simulink model "first"  (R2020b)
settings: Solver=VariableStepAuto  StartTime=0.0  StopTime=10.0  RelTol=1e-3
libraries: vexarmcortexlib x2
settings Model: Creator=Ghost  LastModifiedBy=Ghost

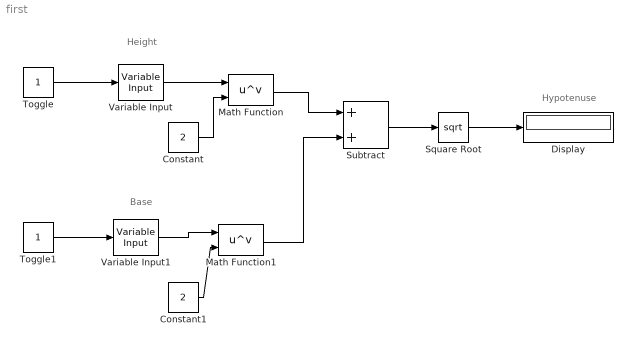
== system first ==
  note: Hypotenuse
  note: Base
  note: Height
  Constant : Constant  Value=2
  Constant1 : Constant  Value=2
  Display : Display
  Math Function : Math  Operator=pow  SignedPower=on  SaturateOnIntegerOverflow=on
  Math Function1 : Math  Operator=pow  SignedPower=on  SaturateOnIntegerOverflow=on
  Square Root : Sqrt  SaturateOnIntegerOverflow=on
  Subtract : Sum
  Toggle : Constant
      settings: OpenFcn=|
      | if strcmp('0',get_param(gcb, 'Value'))                        set_param(gcb, 'Value', '1');
      | else
      |             set_param(gcb, 'Value', '0');
      | end
  Toggle1 : Constant
      settings: OpenFcn=|
      | if strcmp('0',get_param(gcb, 'Value'))                        set_param(gcb, 'Value', '1');
      | else
      |             set_param(gcb, 'Value', '0');
      | end
  Variable Input : vexarmcortexlib/Utilities/Variable Input  low=-127  gain=24  high=127
      settings: SourceProductBaseCode=EC_VEX_MICRO
  Variable Input1 : vexarmcortexlib/Utilities/Variable Input  low=-127  gain=7  high=127
      settings: SourceProductBaseCode=EC_VEX_MICRO
  wires:
  Toggle1/1 -> Variable Input1/1
  Toggle/1 -> Variable Input/1
  Variable Input/1 -> Math Function/1
  Variable Input1/1 -> Math Function1/1
  Math Function1/1 -> Subtract/2
  Math Function/1 -> Subtract/1
  Constant/1 -> Math Function/2
  Constant1/1 -> Math Function1/2
  Subtract/1 -> Square Root/1
  Square Root/1 -> Display/1
